simulink model "houseHeatingSystemWithFuzzyControl"  (R2024b)
settings: Solver=FixedStepAuto  StartTime=0.0  StopTime=3600*24*2  FixedStep=10  MaxStep=50  RelTol=1e-3  AbsTol=1e-3
PreLoadFcn:
  | % FIS for setting a desired temperature
  | desiredHT = readfis('desiredHT.fis');
  | 
  | % FPID
  | GE = 0.6667;
  | GCE = 148.8761;
  | GCU = 1.3478e-05;
  | GU = 0.0363;
  | N = 0.000746309714556118;
  | 
  | fpid = readfis('fpid.fis');
  | 
  | %   Simscape Demo "House Heating System"
  | max_temp = 23;    % Maximum temperature
  | min_temp = 18;     % Minimum temperature
  | % Walls
  | % House length = 30 m
  | lenHouse = 30;
  | % House width = 10 m
  | widHouse = 10;
  | % House height = 4 m
  | htHouse = 4;
  | wallArea = 2*lenHouse*htHouse + 2*widHouse*htHouse;
  | LWall = .2;
  | wallVolume = wallArea * LWall;
  | wallDensity = 1920;     % kg/m^3
  | wallMass = wallVolume * wallDensity;
  | c_wall = 835;           % J/kg/K
  | kWall = 0.038;  % Thermal conductivity [W/m/K]
  | % -------------------------------
  | % Windows
  | % Number of windows = 6
  | numWindows = 6;
  | % Height of windows = 1 m
  | htWindows = 1;
  | % Width of windows = 1 m
  | widWindows = 1;
  | windowArea = numWindows*htWindows*widWindows;
  | LWindow = .01;
  | windowVolume = windowArea * LWindow;
  | windowDensity = 2700;       % kg/m^3
  | windowMass = windowVolume * windowDensity;
  | c_window = 840;             % J/kg/K
  | kWindow = 0.78;             % Thermal conductivity [W/m/K]
  | % -------------------------------
  | % Roof
  | % Roof pitch = 40 deg
  | pitRoof = 40/180/pi;
  | roofArea =  2*(1/cos(pitRoof/2))*widHouse*lenHouse + tan(pitRoof)*widHouse;
  | LRoof = 0.2;
  | roofVolume = roofArea * LRoof;
  | roofDensity = 32;           % Glass fiber
  | roofMass = roofVolume * roofDensity;
  | kRoof = 0.038;              % Thermal conductivity [W/m/K]
  | c_roof = 835;               % J/kg/K
  | % -------------------------------
  | % Convective heat gransfer coefficients (W/M^2/K)
  | h_A_W = 24;         % Air-wall
  | h_W_Atm = 34;       % Wall-atmosphere
  | h_A_Wnd = 25;       % Air-window
  | h_Wnd_Atm = 32;     % Window-atmosphere
  | h_A_R = 12;         % Air-roof
  | h_R_Atm = 38;       % Roof-atmosphere
  | % -------------------------------
  | %Air
  | % Density of air at sea level = 1.2250 kg/m^3
  | densAir = 1.2250;
  | % Air mass inside the house
  | M_air = (lenHouse*widHouse*htHouse+tan(pitRoof)*widHouse*lenHouse)*densAir;
  | c_air = 1005.4;         % cp of air at 273 K [J/(kg*K]
  | % -------------------------------
  | % Heater
  | % The air exiting the heater has a constant temperature which is a heater
  | % property. THeater = 50 deg C
  | THeater = 50;
  | HeaterAirFlow = 1;  % Heater air flow rate [kg/s]
  | % -------------------------------
  | % Cost of electricity
  | % Assume the cost of electricity is $0.09 per kilowatt/hour
  | % Assume all electric energy is transformed to heat energy
  | % 1 kW-hr = 3.6e6 J
  | % cost = $0.09 per 3.6e6 J
  | cost = 0.09/3.6e6;
  | lowCost = 0.025; % $/kWh
  | highCost = 0.14; % $/kWh
  | % -------------------------------
  | % Initial internal temperatures
  | TinIC = 20; % deg C
  | % Outdoor temperature settings
  | sinePhase = 0;
  | sineAmplitude = 4;
  | sineBias = 8;
  | sineFreq = 2*pi/(48*3600);
  | TemperatureSampleTime = 300; % 5 minutes
  | % ---- Comfort zone ----
  | T_comfort_min = 20; % deg C
  | T_comfort_max = 22; % deg C
libraries: fl_lib x22, nesl_utility x4, fuzblock x2
CloseFcn:
  | % Desired house temperature FIS
  | clear desiredHT
  | 
  | % FPID
  | clear fpid GE GCE GCU GU N
  | 
  | % Heating system
  | try
  |     close(h1_ssc_house_heating_system)
  | catch
  | end
  | 
  | try
  |     close(h2_ssc_house_heating_system)
  | catch
  | end
  | clear h1_ssc_house_heating_system h2_ssc_house_heating_system ...
  |     simlog_ssc_house_heating_system ...
  |     HeaterAirFlow THeater c_window h_A_Wnd htWindows max_temp roofArea ...
  |     sineBias wallMass windowDensity LRoof TinIC cost h_R_Atm kRoof min_temp ...
  |     roofDensity sineFreq wallVolume windowMass LWall c_air densAir h_W_Atm ...
  |     kWall numWindows roofMass sinePhase widHouse windowVolume LWindow c_roof ...
  |     h_A_R h_Wnd_Atm kWindow roofVolume wallArea widWindows M_air c_wall ...
  |     h_A_W htHouse lenHouse pitRoof sineAmplitude wallDensity windowArea ...
  |     TemperatureSampleTime lowCost highCost T_comfort_min T_comfort_max
Description:
  | House Heating System
settings Model: Creator=The MathWorks, Inc.  LastModifiedBy=Tech Assignment 02
settings SolverCC: AutoScaleAbsTol=off  AlgebraicLoopSolver=TrustRegion
settings DataIOCC: ExternalInput=[]  InitialState=[]  SaveFormat=StructureWithTime  SaveOutput=off  SignalLogging=off  DSMLogging=off  SaveTime=off  ReturnWorkspaceOutputs=off  SignalLoggingName=househeat_output  DatasetSignalFormat=timetable
settings OptimizationCC: BlockReduction=off  BooleanDataType=off  ReuseModelBlockBuffer=off  ExpressionDepthLimit=2147483647  InitFltsAndDblsToZero=on  LifeSpan=inf  BufferReusableBoundary=off
settings DebuggingCC: SaveWithParameterizedLinksMsg=none  SignalResolutionControl=TryResolveAllWithWarning  MultiTaskDSMMsg=warning  MultiTaskCondExecSysMsg=none  IntegerOverflowMsg=none  UnconnectedInputMsg=warning  UnconnectedOutputMsg=warning  UnconnectedLineMsg=warning  BusObjectLabelMismatch=none  AllowSymbolicDim=off  StateNameClashWarn=warning  PregeneratedLibrarySubsystemCodeDiagnostic=none  SubsystemReferenceDiagnosticForUnitTest=warning  SFUnexpectedBacktrackingDiag=warning  SFNoUnconditionalDefaultTransitionDiag=warning  SFExecutionAtInitializationDiag=none  IntegerSaturationMsg=none  ArithmeticOperatorsInVariantConditions=warning
settings HardwareCC: ProdBitPerPointer=32  ProdBitPerSizeT=32  ProdBitPerPtrDiffT=32  ProdLargestAtomicFloat=None  ProdIntDivRoundTo=Undefined  ProdEndianess=Unspecified  ProdWordSize=32  ProdHWDeviceType=32-bit Generic  TargetUnknown=on
settings ModelReferenceCC: EnableRefExpFcnMdlSchedulingChecks=on  PropagateSignalLabelsOutOfModel=off
settings SFSimCC: SimUseLocalCustomCode=off  SimParseCustomCode=off  CustomCodeUndefinedFunction=UseInterfaceOnly
settings RTWCC: RTWUseLocalCustomCode=off  GPUComputeCapability=3.5  DLArmComputeVersion=19.05
settings CodeAppCC: StateflowObjectComments=on
settings GRTTargetCC: TargetFcnLib=ansi_tfl_tmw.mat  TargetLangStandard=C89/C90 (ANSI)  CombineOutputUpdateFcns=off  GRTInterface=on
settings ConfigComp: CovMetricSettings=dw  CovSaveCumulativeToWorkspaceVar=on  CovSaveSingleToWorkspaceVar=on  CovExternalEMLEnable=off  CovSFcnEnable=off
settings SimscapeCC: SimscapeLogType=all  SimscapeLogSimulationStatistics=on  SimscapeLogName=simlog_ssc_house_heating_system  SimscapeLogDataHistory=25000

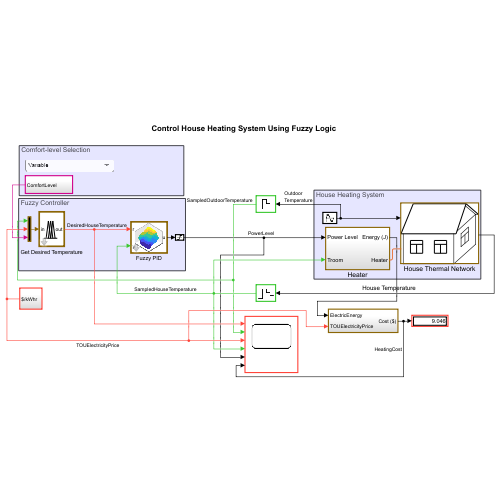
[thumbnail: Simulink's stored preview of the top-level diagram]
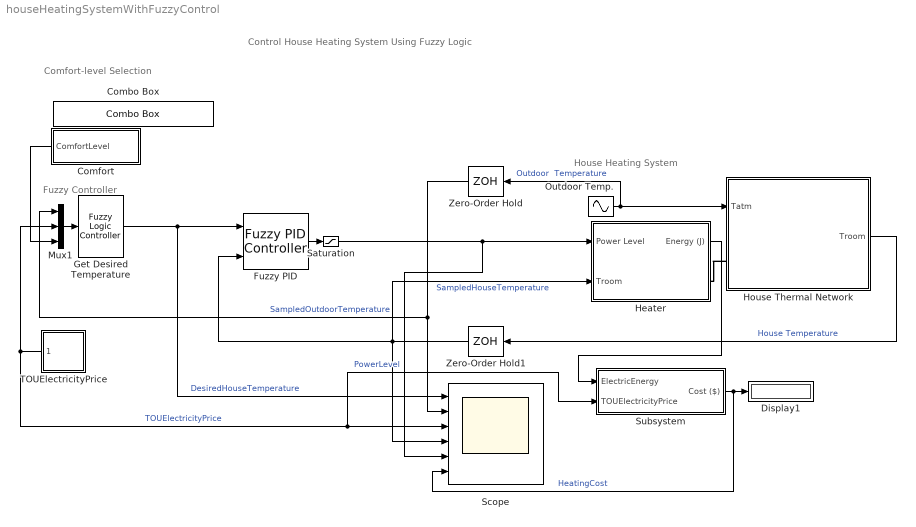
== system houseHeatingSystemWithFuzzyControl ==
  note: Comfort-level Selection
  note: Fuzzy Controller
  note: House Heating System
  note: Control House Heating System Using Fuzzy Logic
  Combo Box : ComboBox  LabelPosition=Hide  SelectedLabel=Variable
      settings: Values={{'Minimum', 'Variable', 'Maximum'}, [1 2 3]}
  Comfort : Subsystem
  Display1 : Display
  Fuzzy PID : fuzblock/Fuzzy PID Controller  TimeDomainType=Continuous-time  CE=GE  CD=GCE  C0=GCU  C1=GU  UseAccumulator=on  IntegratorMethod=Forward Euler  DerivativeSignal=Error (e)  UseFilter=on  N=N  DerivativeFilterMethod=Forward Euler  AddFFRefIn=off  E=off  SampleTime=-1  FIS=fpid  OutputSampleNumber=101  UseLookupTable=off  NumBreakpoints=10
  Get Desired Temperature : fuzblock/Fuzzy Logic  Controller  FIS=desiredHT  OutputSampleNumber=101  DataType=double  FuzzifiedInputs=off  RuleFiringStrengths=off  RuleOutputs=off  AggregatedOutputs=off  SimulateUsing=Interpreted execution  OutOfRangeInputValueMessage=warning  NoRuleFiredMessage=warning  EmptyOutputFuzzySetMessage=warning
  Heater : Subsystem
  House Thermal Network : Subsystem  Tag=PublishSubsystem
      mask Display:
      | plot([99.4454661849886;170.309218810871;170.309218810871;99.4454661849886;99.4454661849886], [212.827470386401;212.827470386401;127.790967235342;127.790967235342;212.827470386401])
      | plot([99.4454661849886;170.309218810871], [184.481969336048;184.481969336048])
      | plot([133.460067445412;133.460067445412], [184.481969336048;127.790967235342])
      | plot([241.172971436754;312.036724062636;312.036724062636;241.172971436754;241.172971436754], [212.827470386401;212.827470386401;127.790967235342;127.790967235342;212.827470386401])
      | plot([241.172971436754;312.036724062636], [184.481969336048;184.481969336048])
      | plot([275.187572697178;275.187572697178], [184.481969336048;127.790967235342])
      | plot([113.618216710165;42.7544640842825;368.727726163343;428.253278369084], [453.764229314402;255.34572196193;255.34572196193;453.764229314402])
      | plot([428.253278369084;499.117030994967], [453.764229314402;382.900476688519])
      | plot([113.618216710165;428.253278369084], [453.764229314402;453.764229314402])
      | plot([498.86507098563;499.368991004303], [382.900476688519;382.900476688519])
      | plot([482.109730364755;496.282480889931], [382.900476688519;382.900476688519])
      | plot([482.109730364755;374.396826373413], [382.900476688519;275.187572697178])
      | plot([482.109730364755;425.418728264049], [382.900476688519;439.591478789225])
      | plot([56.927214609459;56.927214609459;354.554975638166], [255.34572196193;56.927214609459;56.927214609459])
      | plot([354.554975638166;354.554975638166], [56.927214609459;255.34572196193])
      | plot([354.554975638166;482.109730364755;482.109730364755], [56.927214609459;184.481969336048;382.900476688519])
      | plot([397.073227213696;397.073227213696;439.591478789225;439.591478789225;397.073227213696], [170.309218810871;255.34572196193;297.86397353746;209.992920281366;170.309218810871])
      | plot([397.073227213696;439.591478789225], [227.000220911577;269.518472487107])
      | plot([419.749628053978;419.749628053978], [246.842071646824;192.985619651154])
      | %patch([0;553.20969549939;553.20969549939;0;0;0.472425017505884;0.47242501750577;552.737270481884;552.737270481885;0.472425017505884;0], [496.518693398684;496.518693398684;0;0;496.518693398684;496.046268381178;0.472425017505884;0.472425017505884;496.046268381178;496.046268381178;496.518693398684], [1;1;1])
  Mux1 : Mux  Inputs=3
  Outdoor Temp. : Sin  Amplitude=sineAmplitude  Bias=sineBias  Frequency=sineFreq  Phase=sinePhase  SampleTime=0
  Saturation : Saturate  UpperLimit=1  LowerLimit=0
  Scope : Scope  NumInputPorts=6
  Subsystem : Subsystem
  TOUElectricityPrice : Subsystem
  Zero-Order Hold : ZeroOrderHold  SampleTime=TemperatureSampleTime
  Zero-Order Hold1 : ZeroOrderHold  SampleTime=TemperatureSampleTime
  wires:
  House Thermal Network/1(Troom) -> Zero-Order Hold1/1  "House Temperature"
  Outdoor Temp./1 -> Zero-Order Hold/1, House Thermal Network/1(Tatm)  "Outdoor  Temperature"
  Zero-Order Hold1/1 -> Scope/4, Fuzzy PID/2, Heater/2(Troom)  "SampledHouseTemperature"
  Fuzzy PID/1 -> Saturation/1
  Saturation/1 -> Scope/5, Heater/1(Power Level)  "PowerLevel"
  Zero-Order Hold/1 -> Mux1/1, Scope/2  "SampledOutdoorTemperature"
  Mux1/1 -> Get Desired Temperature/1
  TOUElectricityPrice/1($/kWhr) -> Mux1/2, Subsystem/2(TOUElectricityPrice), Scope/3  "TOUElectricityPrice"
  Subsystem/1(Cost ($)) -> Scope/6, Display1/1  "HeatingCost"
  Get Desired Temperature/1 -> Scope/1, Fuzzy PID/1  "DesiredHouseTemperature"
  Heater/1(Energy (J)) -> Subsystem/1(ElectricEnergy)
  Comfort/1(ComfortLevel) -> Mux1/3
  connections:
  House Thermal Network/LConn1 -- Heater/RConn1

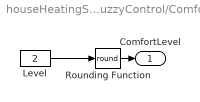
== system houseHeatingSystemWithFuzzyControl/Comfort ==
  Level : Constant  Value=2  OutMin=1  OutMax=3
  Rounding Function : Rounding  Operator=round
  ComfortLevel : Outport
  wires:
  Level/1 -> Rounding Function/1
  Rounding Function/1 -> ComfortLevel/1

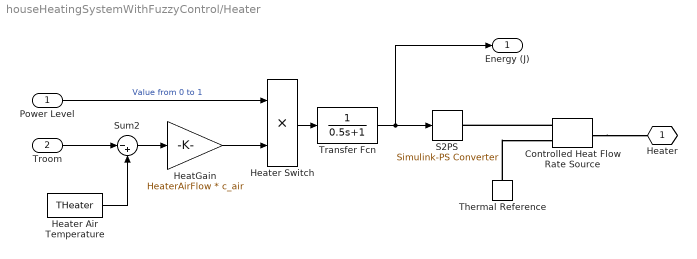
== system houseHeatingSystemWithFuzzyControl/Heater ==
  Power Level : Inport
  Troom : Inport  Port=2
  Controlled Heat Flow Rate Source : fl_lib/Thermal/Thermal Sources/Controlled Heat Flow Rate Source
  HeatGain : Gain  Gain=HeaterAirFlow * c_air
  Heater Air Temperature : Constant  Value=THeater
  Heater Switch : Product  RndMeth=Zero
  S2PS : nesl_utility/Simulink-PS Converter  PhysicalDomain=network_engine_domain  SubClassName=ps_input  LeftPortType=input  RightPortType=output  PseudoPeriodic=off  Frequencies=[]  NoiseDistribution=none  NoiseParameters=[]  Unit=1  AffineConversion=off  FilteringAndDerivatives=zero  SimscapeFilterOrder=1  InputFilterTimeConstant=.001  UdotUserProvided=0
  Sum2 : Sum  Inputs=|-+
  Thermal Reference : fl_lib/Thermal/Thermal Elements/Thermal Reference
  Transfer Fcn : TransferFcn  Denominator=[0.5 1]
  Heater : PMIOPort  Tag=PMCPort  Side=Right
  Energy (J) : Outport
  wires:
  Heater Air Temperature/1 -> Sum2/2
  Troom/1 -> Sum2/1
  Sum2/1 -> HeatGain/1
  Power Level/1 -> Heater Switch/1  "Value from 0 to 1"
  HeatGain/1 -> Heater Switch/2
  Heater Switch/1 -> Transfer Fcn/1
  Transfer Fcn/1 -> Energy (J)/1, S2PS/1
  connections:
  Controlled Heat Flow Rate Source/RConn1 -- S2PS/RConn1
  Thermal Reference/LConn1 -- Controlled Heat Flow Rate Source/RConn2
  Controlled Heat Flow Rate Source/LConn1 -- Heater/RConn1

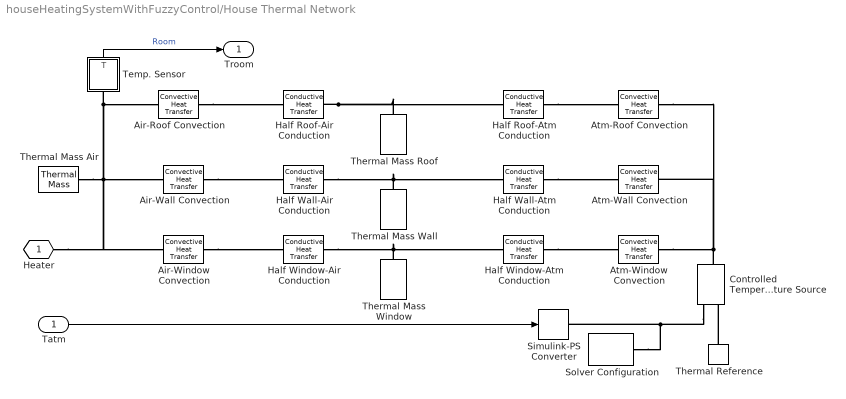
== system houseHeatingSystemWithFuzzyControl/House Thermal Network ==
  Tatm : Inport
  Air-Roof Convection : fl_lib/Thermal/Thermal Elements/Convective Heat Transfer  thermal_type=foundation.enum.constant_variable.constant  area=roofArea m^2  heat_tr_coeff=h_A_R W/m^2/K  min_heat_tr_coeff=1e-3 W/(K*m^2)  T_specify=off  T_priority=High  T=0 K  T_nominal_specify=off  T_nominal_value=1  T_nominal_unit=K  Q_specify=off  Q_priority=High  Q=0 J/s  Q_nominal_specify=off  Q_nominal_value=1  Q_nominal_unit=W
  Air-Wall Convection : fl_lib/Thermal/Thermal Elements/Convective Heat Transfer  thermal_type=foundation.enum.constant_variable.constant  area=wallArea m^2  heat_tr_coeff=h_A_W W/m^2/K  min_heat_tr_coeff=1e-3 W/(K*m^2)  T_specify=off  T_priority=High  T=0 K  T_nominal_specify=off  T_nominal_value=1  T_nominal_unit=K  Q_specify=off  Q_priority=High  Q=0 J/s  Q_nominal_specify=off  Q_nominal_value=1  Q_nominal_unit=W
  Air-Window Convection : fl_lib/Thermal/Thermal Elements/Convective Heat Transfer  thermal_type=foundation.enum.constant_variable.constant  area=windowArea m^2  heat_tr_coeff=h_A_Wnd W/m^2/K  min_heat_tr_coeff=1e-3 W/(K*m^2)  T_specify=off  T_priority=High  T=0 K  T_nominal_specify=off  T_nominal_value=1  T_nominal_unit=K  Q_specify=off  Q_priority=High  Q=0 J/s  Q_nominal_specify=off  Q_nominal_value=1  Q_nominal_unit=W
  Atm-Roof Convection : fl_lib/Thermal/Thermal Elements/Convective Heat Transfer  thermal_type=foundation.enum.constant_variable.constant  area=roofArea m^2  heat_tr_coeff=h_R_Atm W/m^2/K  min_heat_tr_coeff=1e-3 W/(K*m^2)  T_specify=off  T_priority=High  T=0 K  T_nominal_specify=off  T_nominal_value=1  T_nominal_unit=K  Q_specify=off  Q_priority=High  Q=0 J/s  Q_nominal_specify=off  Q_nominal_value=1  Q_nominal_unit=W
  Atm-Wall Convection : fl_lib/Thermal/Thermal Elements/Convective Heat Transfer  thermal_type=foundation.enum.constant_variable.constant  area=wallArea m^2  heat_tr_coeff=h_W_Atm W/m^2/K  min_heat_tr_coeff=1e-3 W/(K*m^2)  T_specify=off  T_priority=High  T=0 K  T_nominal_specify=off  T_nominal_value=1  T_nominal_unit=K  Q_specify=off  Q_priority=High  Q=0 J/s  Q_nominal_specify=off  Q_nominal_value=1  Q_nominal_unit=W
  Atm-Window Convection : fl_lib/Thermal/Thermal Elements/Convective Heat Transfer  thermal_type=foundation.enum.constant_variable.constant  area=windowArea m^2  heat_tr_coeff=h_Wnd_Atm W/m^2/K  min_heat_tr_coeff=1e-3 W/(K*m^2)  T_specify=off  T_priority=High  T=0 K  T_nominal_specify=off  T_nominal_value=1  T_nominal_unit=K  Q_specify=off  Q_priority=High  Q=0 J/s  Q_nominal_specify=off  Q_nominal_value=1  Q_nominal_unit=W
  Controlled Temperature Source : fl_lib/Thermal/Thermal Sources/Controlled Temperature Source
  Half Roof-Air Conduction : fl_lib/Thermal/Thermal Elements/Conductive Heat Transfer  thermal_type=foundation.enum.ConstantVariableTabulated.Constant  wall_geometry=foundation.enum.ConductionWallGeometry.Planar  area=roofArea m^2  thickness=LRoof/2 m  d_in=0.05 m  d_out=0.1 m  L=1 m  th_cond_min=10 W/(K*m)  th_cond=kRoof W/m/K  th_cond_TLU=[413, 401, 392, 383, 371, 357, 342] W/(K*m)  temp_TLU=[200, 273, 400, 600, 800, 1000, 1200] K  T_specify=off  T_priority=High  T=0 K  T_nominal_specify=off  T_nominal_value=1  T_nominal_unit=K  Q_specify=off  Q_priority=High  Q=0 J/s  Q_nominal_specify=off  Q_nominal_value=1  Q_nominal_unit=W
  Half Roof-Atm Conduction : fl_lib/Thermal/Thermal Elements/Conductive Heat Transfer  thermal_type=foundation.enum.ConstantVariableTabulated.Constant  wall_geometry=foundation.enum.ConductionWallGeometry.Planar  area=roofArea m^2  thickness=LRoof/2 m  d_in=0.05 m  d_out=0.1 m  L=1 m  th_cond_min=10 W/(K*m)  th_cond=kRoof W/m/K  th_cond_TLU=[413, 401, 392, 383, 371, 357, 342] W/(K*m)  temp_TLU=[200, 273, 400, 600, 800, 1000, 1200] K  T_specify=off  T_priority=High  T=0 K  T_nominal_specify=off  T_nominal_value=1  T_nominal_unit=K  Q_specify=off  Q_priority=High  Q=0 J/s  Q_nominal_specify=off  Q_nominal_value=1  Q_nominal_unit=W
  Half Wall-Air Conduction : fl_lib/Thermal/Thermal Elements/Conductive Heat Transfer  thermal_type=foundation.enum.ConstantVariableTabulated.Constant  wall_geometry=foundation.enum.ConductionWallGeometry.Planar  area=wallArea m^2  thickness=LWall/2 m  d_in=0.05 m  d_out=0.1 m  L=1 m  th_cond_min=10 W/(K*m)  th_cond=kWall W/m/K  th_cond_TLU=[413, 401, 392, 383, 371, 357, 342] W/(K*m)  temp_TLU=[200, 273, 400, 600, 800, 1000, 1200] K  T_specify=off  T_priority=High  T=0 K  T_nominal_specify=off  T_nominal_value=1  T_nominal_unit=K  Q_specify=off  Q_priority=High  Q=0 J/s  Q_nominal_specify=off  Q_nominal_value=1  Q_nominal_unit=W
  Half Wall-Atm Conduction : fl_lib/Thermal/Thermal Elements/Conductive Heat Transfer  thermal_type=foundation.enum.ConstantVariableTabulated.Constant  wall_geometry=foundation.enum.ConductionWallGeometry.Planar  area=wallArea m^2  thickness=LWall/2 m  d_in=0.05 m  d_out=0.1 m  L=1 m  th_cond_min=10 W/(K*m)  th_cond=kWall W/m/K  th_cond_TLU=[413, 401, 392, 383, 371, 357, 342] W/(K*m)  temp_TLU=[200, 273, 400, 600, 800, 1000, 1200] K  T_specify=off  T_priority=High  T=0 K  T_nominal_specify=off  T_nominal_value=1  T_nominal_unit=K  Q_specify=off  Q_priority=High  Q=0 J/s  Q_nominal_specify=off  Q_nominal_value=1  Q_nominal_unit=W
  Half Window-Air Conduction : fl_lib/Thermal/Thermal Elements/Conductive Heat Transfer  thermal_type=foundation.enum.ConstantVariableTabulated.Constant  wall_geometry=foundation.enum.ConductionWallGeometry.Planar  area=windowArea m^2  thickness=LWindow/2 m  d_in=0.05 m  d_out=0.1 m  L=1 m  th_cond_min=10 W/(K*m)  th_cond=kWindow W/m/K  th_cond_TLU=[413, 401, 392, 383, 371, 357, 342] W/(K*m)  temp_TLU=[200, 273, 400, 600, 800, 1000, 1200] K  T_specify=off  T_priority=High  T=0 K  T_nominal_specify=off  T_nominal_value=1  T_nominal_unit=K  Q_specify=off  Q_priority=High  Q=0 J/s  Q_nominal_specify=off  Q_nominal_value=1  Q_nominal_unit=W
  Half Window-Atm Conduction : fl_lib/Thermal/Thermal Elements/Conductive Heat Transfer  thermal_type=foundation.enum.ConstantVariableTabulated.Constant  wall_geometry=foundation.enum.ConductionWallGeometry.Planar  area=windowArea m^2  thickness=LWindow/2 m  d_in=0.05 m  d_out=0.1 m  L=1 m  th_cond_min=10 W/(K*m)  th_cond=kWindow W/m/K  th_cond_TLU=[413, 401, 392, 383, 371, 357, 342] W/(K*m)  temp_TLU=[200, 273, 400, 600, 800, 1000, 1200] K  T_specify=off  T_priority=High  T=0 K  T_nominal_specify=off  T_nominal_value=1  T_nominal_unit=K  Q_specify=off  Q_priority=High  Q=0 J/s  Q_nominal_specify=off  Q_nominal_value=1  Q_nominal_unit=W
  Simulink-PS Converter : nesl_utility/Simulink-PS Converter  PhysicalDomain=network_engine_domain  SubClassName=ps_input  LeftPortType=input  RightPortType=output  PseudoPeriodic=off  Frequencies=[]  NoiseDistribution=none  NoiseParameters=[]  Unit=degC  AffineConversion=on  FilteringAndDerivatives=zero  SimscapeFilterOrder=1  InputFilterTimeConstant=.001  UdotUserProvided=0
  Solver Configuration : nesl_utility/Solver Configuration  PhysicalDomain=network_engine_domain  SubClassName=solver  LeftPortType=input  RightPortType=generic  Tones=[]  Harmonics=[]  SimulateNoise=off  Profile=off  UseLocalSampling=off  EnableSwitchedLinearOptims=on  FrequencyDomain=off  UseCCode=off  RelTol=0.001  AbsTol=1e-06  MinStep=1e-09  ToWorkspace=off  RevertToSquareIcSolve=off  NumHomotopyIterations=100  PhasorMode=off  PhasorModeNumHarmonics=1  ConsistencySolver=NEWTON_XTOL_AFTER_FTOL  IndexReductionMethod=DerivativeReplacement  DoDC=off  ResidualTolerance=1e-9  ConsistencyTolSource=GLOBAL  ConsistencyAbsTol=0.001  ConsistencyRelTol=0.001  ConsistencyTolFactor=0.001  UseLocalSolver=off  LocalSolverChoice=NE_BACKWARD_EULER_ADVANCER  ResolveIndetEquations=on  FunctionEvalNumThread=1  LocalSolverSampleTime=.001  DoFixedCost=off  MaxNonlinIter=3  MaxModeIter=2  ComputeImpulses=off  ImpulseIterations=2  LinearAlgebra=auto  LinearAlgebraNumThread=0  EquationFormulation=NE_TIME_EF  DelaysMemoryBudget=1024  AutomaticFiltering=on  FilteringTimeConstant=0.001  PartitionStorageMethod=AS_NEEDED  PartitionMemoryBudget=1024  PartitionMethod=FAST  MultibodyUseLocalSolver=off  MultibodyLocalSolverChoice=ODE1  MultibodyLocalSolverSampleTime=0.001
  Temp. Sensor : Subsystem
  Thermal Mass Air : fl_lib/Thermal/Thermal Elements/Thermal Mass  mass_type=foundation.enum.constant_variable.constant  mass=M_air kg  sp_heat=c_air J/kg/K  mass_min=1e-6 kg  num_ports=foundation.enum.numPorts2.one  m_specify=off  m_priority=High  m=1 kg  m_nominal_specify=off  m_nominal_value=1  m_nominal_unit=kg  T_specify=on  T_priority=High  T=TinIC degC  T_nominal_specify=off  T_nominal_value=1  T_nominal_unit=K  Q_specify=off  Q_priority=None  Q=0 W  Q_nominal_specify=off  Q_nominal_value=1  Q_nominal_unit=W
  Thermal Mass Roof : fl_lib/Thermal/Thermal Elements/Thermal Mass  mass_type=foundation.enum.constant_variable.constant  mass=roofMass kg  sp_heat=c_roof J/kg/K  mass_min=1e-6 kg  num_ports=foundation.enum.numPorts2.one  m_specify=off  m_priority=High  m=1 kg  m_nominal_specify=off  m_nominal_value=1  m_nominal_unit=kg  T_specify=on  T_priority=High  T=TinIC degC  T_nominal_specify=off  T_nominal_value=1  T_nominal_unit=K  Q_specify=off  Q_priority=None  Q=0 W  Q_nominal_specify=off  Q_nominal_value=1  Q_nominal_unit=W
  Thermal Mass Wall : fl_lib/Thermal/Thermal Elements/Thermal Mass  mass_type=foundation.enum.constant_variable.constant  mass=wallMass kg  sp_heat=c_wall J/kg/K  mass_min=1e-6 kg  num_ports=foundation.enum.numPorts2.one  m_specify=off  m_priority=High  m=1 kg  m_nominal_specify=off  m_nominal_value=1  m_nominal_unit=kg  T_specify=on  T_priority=High  T=TinIC degC  T_nominal_specify=off  T_nominal_value=1  T_nominal_unit=K  Q_specify=off  Q_priority=None  Q=0 W  Q_nominal_specify=off  Q_nominal_value=1  Q_nominal_unit=W
  Thermal Mass Window : fl_lib/Thermal/Thermal Elements/Thermal Mass  mass_type=foundation.enum.constant_variable.constant  mass=windowMass kg  sp_heat=c_window J/kg/K  mass_min=1e-6 kg  num_ports=foundation.enum.numPorts2.one  m_specify=off  m_priority=High  m=1 kg  m_nominal_specify=off  m_nominal_value=1  m_nominal_unit=kg  T_specify=on  T_priority=High  T=TinIC degC  T_nominal_specify=off  T_nominal_value=1  T_nominal_unit=K  Q_specify=off  Q_priority=None  Q=0 W  Q_nominal_specify=off  Q_nominal_value=1  Q_nominal_unit=W
  Thermal Reference : fl_lib/Thermal/Thermal Elements/Thermal Reference
  Heater : PMIOPort  Tag=PMCPort  Side=Left
  Troom : Outport  VectorParamsAs1DForOutWhenUnconnected=off
  wires:
  Tatm/1 -> Simulink-PS Converter/1
  Temp. Sensor/1(T) -> Troom/1  "Room"
  connections:
  Thermal Reference/LConn1 -- Controlled Temperature Source/RConn2
  Solver Configuration/RConn1 -- Controlled Temperature Source/RConn1 -- Simulink-PS Converter/RConn1
  Heater/RConn1 -- Air-Window Convection/LConn1 -- Thermal Mass Air/LConn1 -- Air-Wall Convection/LConn1 -- Air-Roof Convection/LConn1 -- Temp. Sensor/LConn1
  Air-Wall Convection/RConn1 -- Half Wall-Air Conduction/LConn1
  Half Wall-Air Conduction/RConn1 -- Thermal Mass Wall/LConn1 -- Half Wall-Atm Conduction/LConn1
  Half Wall-Atm Conduction/RConn1 -- Atm-Wall Convection/LConn1
  Air-Window Convection/RConn1 -- Half Window-Air Conduction/LConn1
  Half Window-Air Conduction/RConn1 -- Thermal Mass Window/LConn1 -- Half Window-Atm Conduction/LConn1
  Half Window-Atm Conduction/RConn1 -- Atm-Window Convection/LConn1
  Air-Roof Convection/RConn1 -- Half Roof-Air Conduction/LConn1
  Half Roof-Air Conduction/RConn1 -- Half Roof-Atm Conduction/LConn1 -- Thermal Mass Roof/LConn1
  Half Roof-Atm Conduction/RConn1 -- Atm-Roof Convection/LConn1
  Atm-Window Convection/RConn1 -- Controlled Temperature Source/LConn1 -- Atm-Roof Convection/RConn1 -- Atm-Wall Convection/RConn1

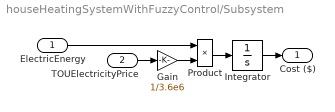
== system houseHeatingSystemWithFuzzyControl/Subsystem ==
  ElectricEnergy : Inport
  TOUElectricityPrice : Inport  Port=2
  Gain : Gain  Gain=1/3.6e6
  Integrator : Integrator
  Product : Product
  Cost ($) : Outport
  wires:
  Product/1 -> Integrator/1
  TOUElectricityPrice/1 -> Gain/1
  Integrator/1 -> Cost ($)/1
  ElectricEnergy/1 -> Product/1
  Gain/1 -> Product/2

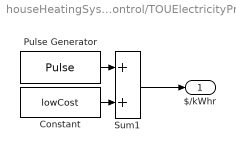
== system houseHeatingSystemWithFuzzyControl/TOUElectricityPrice ==
  Constant : Constant  Value=lowCost
  Pulse Generator : DiscretePulseGenerator  PulseType=Time based  Amplitude=highCost-lowCost  Period=21*3600  PulseWidth=11*100/21  PhaseDelay=10*3600
  Sum1 : Sum
  $/kWhr : Outport
  wires:
  Constant/1 -> Sum1/2
  Pulse Generator/1 -> Sum1/1
  Sum1/1 -> $/kWhr/1

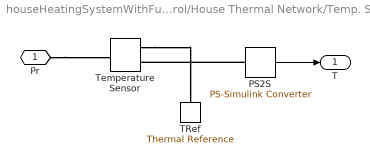
== system houseHeatingSystemWithFuzzyControl/House Thermal Network/Temp. Sensor ==
  PS2S : nesl_utility/PS-Simulink Converter  PhysicalDomain=network_engine_domain  SubClassName=ps_output  LeftPortType=input  RightPortType=output  PseudoPeriodic=off  Frequencies=[]  VectorFormat=1-D array  Unit=degC  AffineConversion=on
  TRef : fl_lib/Thermal/Thermal Elements/Thermal Reference
  Temperature Sensor : fl_lib/Thermal/Thermal Sensors/Temperature Sensor  temperature_measure=foundation.enum.MeasurementReference.difference
  Pr : PMIOPort  Side=Left
  T : Outport  VectorParamsAs1DForOutWhenUnconnected=off
  wires:
  PS2S/1 -> T/1
  connections:
  Temperature Sensor/RConn1 -- TRef/LConn1
  PS2S/LConn1 -- Temperature Sensor/RConn2
  Pr/RConn1 -- Temperature Sensor/LConn1
